simulink model "DownSamplingDemo"  (Simulink 6.3)
settings: Solver=ode45  StartTime=0.0  StopTime=70  RelTol=1e-3
InitFcn:
  | %% DSPBuilder Start
  | alt_dspbuilder_update_model(bdroot)
  | %% DSPBuilder End
libraries: allblocks_alteradspbuilder2 x5
settings Model: LastModifiedBy=delphick
settings OptimizationCC: BlockReduction=off  BooleanDataType=off  InlineInvariantSignals=on
settings DebuggingCC: SolverPrmCheckMsg=none
settings HardwareCC: TargetUnknown=on

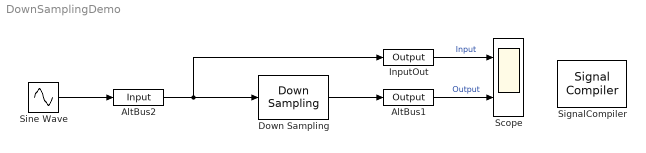
== system DownSamplingDemo ==
  AltBus1 : allblocks_alteradspbuilder2/Output  iofile=C:\workspace_clean\Documentation\DesignExamples\Tutorials\UnitBlocks\Storage\DownSampling\tb_DownSamplingDemo\DownSamplingDemo_AltBus1.capture  BusType=Signed Integer  bwl=5  bwr=4  PORTTYPE=Output
  AltBus2 : allblocks_alteradspbuilder2/Input  iofile=C:\workspace_clean\Documentation\DesignExamples\Tutorials\UnitBlocks\Storage\DownSampling\tb_DownSamplingDemo\DownSamplingDemo_AltBus2.salt  BusType=Signed Integer  bwl=5  bwr=4  SpecifyClock=off  PORTTYPE=Input
  Down Sampling : allblocks_alteradspbuilder2/Down Sampling  rate=4
  InputOut : allblocks_alteradspbuilder2/Output  iofile=C:\workspace_clean\Documentation\DesignExamples\Tutorials\UnitBlocks\Storage\DownSampling\tb_DownSamplingDemo\DownSamplingDemo_InputOut.capture  BusType=Signed Integer  bwl=5  bwr=4  PORTTYPE=Output
  Scope : Scope  NumInputPorts=2
      settings: YMin=-10~-10  YMax=10~10
  SignalCompiler : allblocks_alteradspbuilder2/Signal Compiler  DeviceFamily=Stratix IV  DeviceName=AUTO  EnableSignalTap=off  SignalTapDepth=128  UseBoardBlock=off  StpUseDefaultClock=on  StpClock=clock
  Sine Wave : Sin  Amplitude=8  Frequency=0.1  SampleTime=1
  wires:
  AltBus1/1 -> Scope/2  "Output"
  Down Sampling/1 -> AltBus1/1
  Sine Wave/1 -> AltBus2/1
  AltBus2/1 -> Down Sampling/1, InputOut/1
  InputOut/1 -> Scope/1  "Input"
